simulink model "Redresseur_MLI_3Ph_Hysteresis"  (R2018b)
settings: Solver=ode8  StartTime=0.0  StopTime=Ts  FixedStep=1e-6  RelTol=1e-3
undefined symbols (not defined in the file): C, eps_off, eps_on, Im, inverter_matrix, L, R, V
settings Model: Creator=driss  LastModifiedBy=driss
settings DataIOCC: ReturnWorkspaceOutputs=on
settings DebuggingCC: UnconnectedInputMsg=none  UnconnectedOutputMsg=none  UnconnectedLineMsg=none
settings ModelReferenceCC: EnableRefExpFcnMdlSchedulingChecks=off
settings RTWCC: Description=Generic Real-Time Target

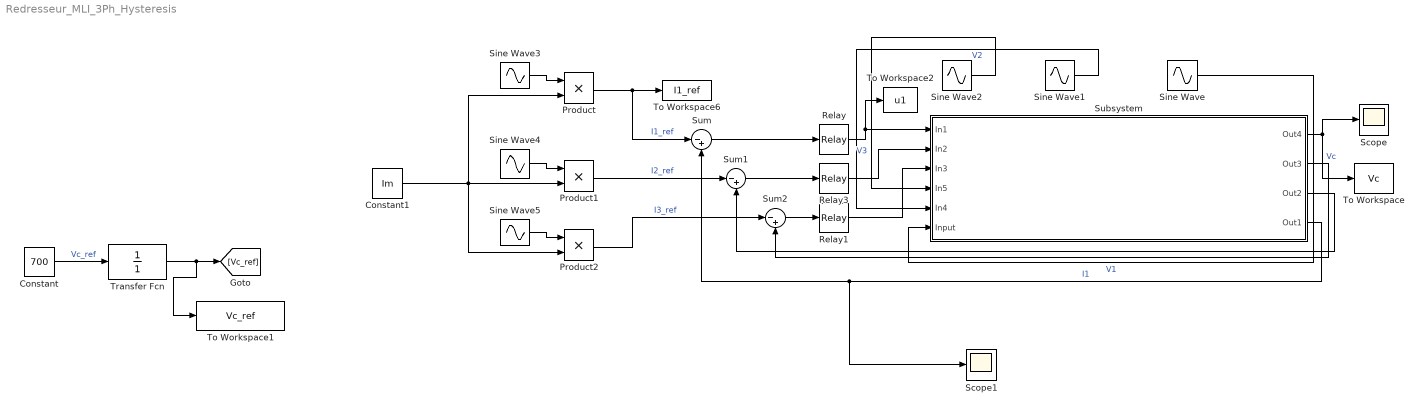
== system Redresseur_MLI_3Ph_Hysteresis ==
  Constant : Constant  Value=700
  Constant1 : Constant  Value=Im
  Product : Product
  Product1 : Product
  Product2 : Product
  Relay : Relay  OnSwitchValue=eps_on  OffSwitchValue=eps_off  OnOutputValue=S_on  OffOutputValue=S_off
  Relay1 : Relay  OnSwitchValue=eps_on  OffSwitchValue=eps_off  OnOutputValue=S_on  OffOutputValue=S_off
  Relay3 : Relay  OnSwitchValue=eps_on  OffSwitchValue=eps_off  OnOutputValue=S_on  OffOutputValue=S_off
  Scope : Scope
  Scope1 : Scope
  Sine Wave : Sin  Amplitude=V*sqrt(2)  Frequency=2*50*pi  SampleTime=0
  Sine Wave1 : Sin  Amplitude=V*sqrt(2)  Frequency=2*50*pi  Phase=-2*pi/3  SampleTime=0
  Sine Wave2 : Sin  Amplitude=V*sqrt(2)  Frequency=2*50*pi  Phase=-4*pi/3  SampleTime=0
  Sine Wave3 : Sin  Frequency=2*50*pi  SampleTime=0
  Sine Wave4 : Sin  Frequency=2*50*pi  Phase=-2*pi/3  SampleTime=0
  Sine Wave5 : Sin  Frequency=2*50*pi  Phase=-4*pi/3  SampleTime=0
  Subsystem : Subsystem
  Sum : Sum  Inputs=|-+
  Sum1 : Sum  Inputs=|-+
  Sum2 : Sum  Inputs=|-+
  To Workspace : ToWorkspace  VariableName=Vc  SaveFormat=Timeseries  SampleTime=-1
  To Workspace1 : ToWorkspace  VariableName=Vc_ref  SaveFormat=Timeseries  SampleTime=-1
  To Workspace2 : ToWorkspace  VariableName=u1  SaveFormat=Timeseries  SampleTime=-1
  To Workspace6 : ToWorkspace  VariableName=I1_ref  SaveFormat=Timeseries  SampleTime=-1
  Transfer Fcn : TransferFcn  Denominator=[1]
  wires:
  Sine Wave/1 -> Subsystem/6(Input)  "V1"
  Sum/1 -> Relay/1
  Sum1/1 -> Relay3/1
  Sum2/1 -> Relay1/1
  Product1/1 -> Sum1/1  "I2_ref"
  Product2/1 -> Sum2/1  "I3_ref"
  Subsystem/1(Out4) -> To Workspace/1, Scope/1  "Vc"
  Subsystem/2(Out3) -> Sum2/2
  Subsystem/3(Out2) -> Sum1/2
  Subsystem/4(Out1) -> Scope1/1, Sum/2  "I1"
  Constant/1 -> Transfer Fcn/1  "Vc_ref"
  Relay3/1 -> Subsystem/2(In2)
  Relay1/1 -> Subsystem/3(In3)
  Relay/1 -> To Workspace2/1, Subsystem/1(In1)
  Constant1/1 -> Product2/2, Product/2, Product1/2
  Sine Wave3/1 -> Product/1
  Sine Wave4/1 -> Product1/1
  Sine Wave5/1 -> Product2/1
  Sine Wave2/1 -> Subsystem/4(In5)  "V3"
  Sine Wave1/1 -> Subsystem/5(In4)  "V2"
  Product/1 -> To Workspace6/1, Sum/1  "I1_ref"
  Transfer Fcn/1 -> To Workspace1/1, [Vc_ref]

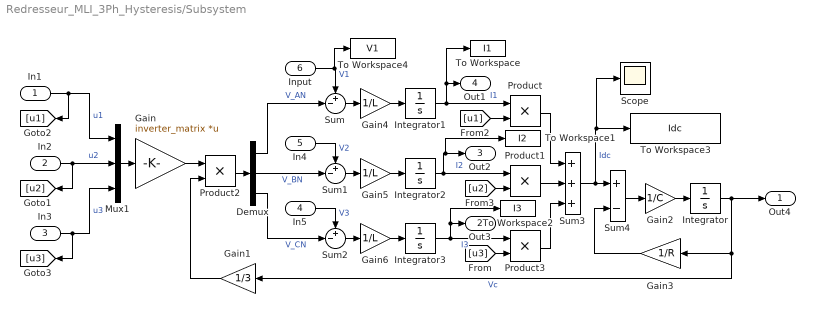
== system Redresseur_MLI_3Ph_Hysteresis/Subsystem ==
  In1 : Inport
  In2 : Inport  Port=2
  In3 : Inport  Port=3
  In5 : Inport  Port=4
  In4 : Inport  Port=5
  Input : Inport  Port=6
  Demux : Demux  Outputs=3
  Gain : Gain  Gain=inverter_matrix  Multiplication=Matrix(K*u)
  Gain1 : Gain  Gain=1/3
  Gain2 : Gain  Gain=1/C
  Gain3 : Gain  Gain=1/R
  Gain4 : Gain  Gain=1/L
  Gain5 : Gain  Gain=1/L
  Gain6 : Gain  Gain=1/L
  Integrator : Integrator  InitialCondition=sqrt(3*2)*V  LowerSaturationLimit=0
  Integrator1 : Integrator
  Integrator2 : Integrator
  Integrator3 : Integrator
  Mux1 : Mux  Inputs=3
  Product{,1..3} (4 alike) : Product
  Scope : Scope
  Sum : Sum  Inputs=+-|
  Sum1 : Sum  Inputs=+-|
  Sum2 : Sum  Inputs=+-|
  Sum3 : Sum  Inputs=+++
  Sum4 : Sum  Inputs=+-
  To Workspace : ToWorkspace  VariableName=I1  SaveFormat=Timeseries  SampleTime=-1
  To Workspace1 : ToWorkspace  VariableName=I2  SaveFormat=Timeseries  SampleTime=-1
  To Workspace2 : ToWorkspace  VariableName=I3  SaveFormat=Timeseries  SampleTime=-1
  To Workspace3 : ToWorkspace  VariableName=Idc  SaveFormat=Timeseries  SampleTime=-1
  To Workspace4 : ToWorkspace  VariableName=V1  SaveFormat=Timeseries  SampleTime=-1
  Out4 : Outport  VectorParamsAs1DForOutWhenUnconnected=on
  Out3 : Outport  Port=2  VectorParamsAs1DForOutWhenUnconnected=on
  Out2 : Outport  Port=3  VectorParamsAs1DForOutWhenUnconnected=on
  Out1 : Outport  Port=4  VectorParamsAs1DForOutWhenUnconnected=on
  wires:
  In3/1 -> [u3], Mux1/3  "u3"
  In2/1 -> [u2], Mux1/2  "u2"
  In1/1 -> [u1], Mux1/1  "u1"
  Demux/2 -> Sum1/2  "V_BN"
  Demux/3 -> Sum2/2  "V_CN"
  Demux/1 -> Sum/2  "V_AN"
  Input/1 -> To Workspace4/1, Sum/1  "V1"
  In4/1 -> Sum1/1  "V2"
  In5/1 -> Sum2/1  "V3"
  Sum/1 -> Gain4/1
  Sum1/1 -> Gain5/1
  Sum2/1 -> Gain6/1
  Integrator1/1 -> To Workspace/1, Out1/1, Product/1  "I1"
  Integrator3/1 -> To Workspace2/1, Out3/1, Product3/1  "I3"
  Integrator2/1 -> Product1/1, To Workspace1/1, Out2/1  "I2"
  Mux1/1 -> Gain/1
  [u3] -> Product3/2
  Product/1 -> Sum3/1
  Product1/1 -> Sum3/2
  Product3/1 -> Sum3/3
  Gain1/1 -> Product2/2
  Gain/1 -> Product2/1
  Sum3/1 -> Scope/1, To Workspace3/1, Sum4/1  "Idc"
  Sum4/1 -> Gain2/1
  Gain2/1 -> Integrator/1
  Integrator/1 -> Out4/1, Gain1/1, Gain3/1  "Vc"
  Gain3/1 -> Sum4/2
  Gain4/1 -> Integrator1/1
  Gain5/1 -> Integrator2/1
  Gain6/1 -> Integrator3/1
  Product2/1 -> Demux/1
  [u1] -> Product/2
  [u2] -> Product1/2
